simulink model "NewtonHeatingCooling_simulink"  (R2016b)
settings: Solver=VariableStepAuto  StartTime=0.0  StopTime=80  RelTol=1e-3
settings Model: Creator=Winxberry  LastModifiedBy=Winxberry

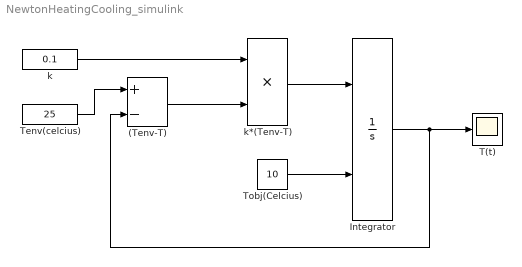
== system NewtonHeatingCooling_simulink ==
  (Tenv-T) : Sum  Inputs=+-
  Integrator : Integrator  InitialConditionSource=external  InitialCondition=100
  T(t) : Scope
  Tenv(celcius) : Constant  Value=25
  Tobj(Celcius) : Constant  Value=10
  k : Constant  Value=0.1
  k*(Tenv-T) : Product
  wires:
  (Tenv-T)/1 -> k*(Tenv-T)/2
  k*(Tenv-T)/1 -> Integrator/1
  k/1 -> k*(Tenv-T)/1
  Tenv(celcius)/1 -> (Tenv-T)/1
  Tobj(Celcius)/1 -> Integrator/2
  Integrator/1 -> (Tenv-T)/2, T(t)/1
